simulink model "P_controller"  (Simulink 7.7)
settings: Solver=ode45  StartTime=0.0  StopTime=L  RelTol=1e-3
values from neighbouring files (symbols this model uses):
  H = 1.5    [main.m]
  Ki = 3    [main.m]
  Kinput = H    (= 1.5)    [main.m]
  Kp = 5    [main.m]
settings Model: Creator=Desktop  LastModifiedBy=Desktop
settings DebuggingCC: SolverPrmCheckMsg=none

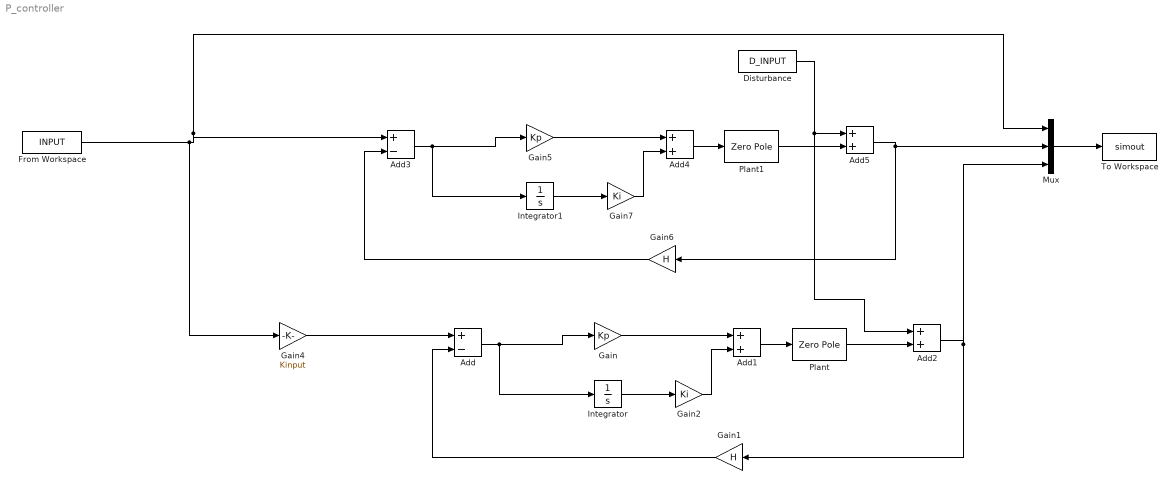
== system P_controller ==
  Add : Sum  Inputs=+-
  Add{1..2,4..5} (4 alike) : Sum
  Add3 : Sum  Inputs=+-
  Disturbance : FromWorkspace  VariableName=D_INPUT  SampleTime=0
  From Workspace : FromWorkspace  VariableName=INPUT  SampleTime=0
  Gain : Gain  Gain=Kp
  Gain1 : Gain  Gain=H
  Gain2 : Gain  Gain=Ki
  Gain4 : Gain  Gain=Kinput
  Gain5 : Gain  Gain=Kp
  Gain6 : Gain  Gain=H
  Gain7 : Gain  Gain=Ki
  Integrator : Integrator
  Integrator1 : Integrator
  Mux : Mux  Inputs=3
  Plant : ZeroPole  Zeros=[0]  Poles=[0 -1]
  Plant1 : ZeroPole  Zeros=[0]  Poles=[0 -1]
  To Workspace : ToWorkspace  VariableName=simout  SampleTime=-1  SaveFormat=Structure
  wires:
  Add/1 -> Gain/1, Integrator/1
  From Workspace/1 -> Mux/1, Add3/1, Gain4/1
  Gain1/1 -> Add/2
  Mux/1 -> To Workspace/1
  Add1/1 -> Plant/1
  Gain/1 -> Add1/1
  Gain2/1 -> Add1/2
  Gain4/1 -> Add/1
  Integrator/1 -> Gain2/1
  Plant/1 -> Add2/2
  Add2/1 -> Gain1/1, Mux/3
  Add3/1 -> Gain5/1, Integrator1/1
  Gain6/1 -> Add3/2
  Add4/1 -> Plant1/1
  Gain5/1 -> Add4/1
  Gain7/1 -> Add4/2
  Integrator1/1 -> Gain7/1
  Plant1/1 -> Add5/2
  Add5/1 -> Gain6/1, Mux/2
  Disturbance/1 -> Add5/1, Add2/1
